simulink model "PMSM_DEE"  (R2023b)
settings: Solver=ode23t  StartTime=0.0  StopTime=0.4  RelTol=1e-3  EnableMultiTasking=on
libraries: powerlib_extras x3, spspowerguiLib x1
settings Model: Creator=Administrator  LastModifiedBy=Guoguo
settings SolverCC: AlgebraicLoopSolver=TrustRegion
settings DataIOCC: LimitDataPoints=on  SaveFormat=Array  SignalLoggingSaveFormat=ModelDataLogs  ReturnWorkspaceOutputs=off
settings OptimizationCC: InitFltsAndDblsToZero=on  LifeSpan=inf
settings DebuggingCC: SaveWithParameterizedLinksMsg=none  UnderspecifiedInitializationDetection=Classic  MergeDetectMultiDrivingBlocksExec=none  SolverPrmCheckMsg=warning  MultiTaskCondExecSysMsg=none  FcnCallInpInsideContextMsg=warning  UnconnectedInputMsg=warning  UnconnectedOutputMsg=warning  UnconnectedLineMsg=warning  SFUnexpectedBacktrackingDiag=warning  SFNoUnconditionalDefaultTransitionDiag=warning  SFExecutionAtInitializationDiag=none  ArithmeticOperatorsInVariantConditions=warning
settings HardwareCC: ProdBitPerPointer=32  ProdBitPerSizeT=32  ProdBitPerPtrDiffT=32  ProdLargestAtomicFloat=None  ProdIntDivRoundTo=Undefined  ProdEndianess=Unspecified  ProdWordSize=32  ProdHWDeviceType=32-bit Generic
settings ModelReferenceCC: PropagateSignalLabelsOutOfModel=off
settings SFSimCC: SimUseLocalCustomCode=off  CustomCodeUndefinedFunction=UseInterfaceOnly
settings RTWCC: RTWUseLocalCustomCode=off
settings CodeAppCC: StateflowObjectComments=on
settings GRTTargetCC: TargetFcnLib=ansi_tfl_tmw.mat  TargetLangStandard=C89/C90 (ANSI)  CombineOutputUpdateFcns=off  GRTInterface=on
settings ConfigComp: CovMetricSettings=dw  CovSaveCumulativeToWorkspaceVar=on  CovSaveSingleToWorkspaceVar=on  CovExternalEMLEnable=off  CovSFcnEnable=off

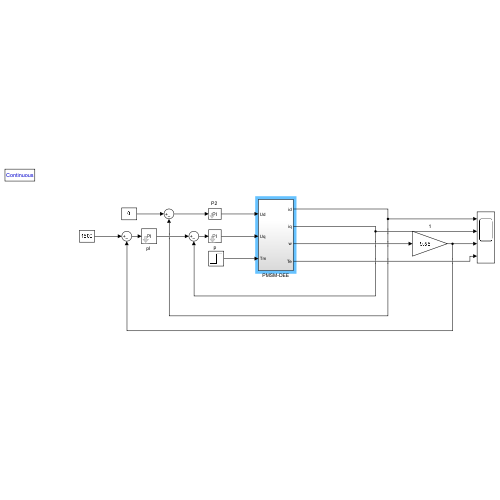
[thumbnail: Simulink's stored preview of the top-level diagram]
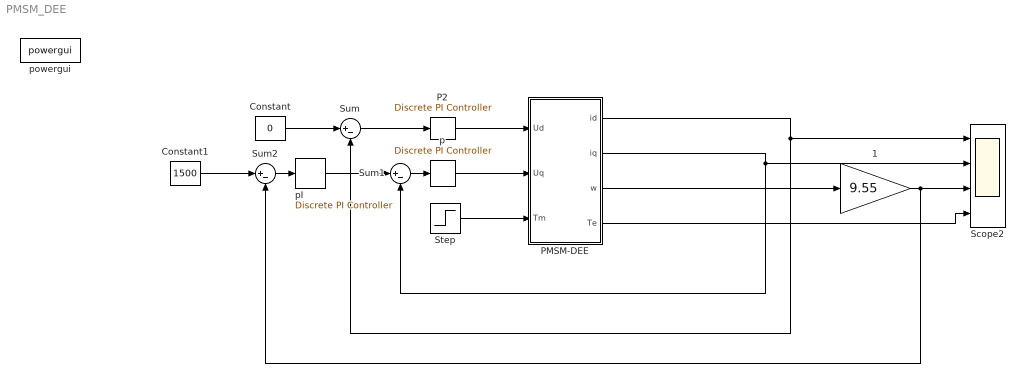
== system PMSM_DEE ==
  1 : Gain  Gain=9.55
  Constant : Constant  Value=0
  Constant1 : Constant  Value=1500
  "P2 " : powerlib_extras/Discrete  Control Blocks/Discrete PI Controller  Kp=21.25  Ki=7187.5  Par_Limits=[250 -250]  Init=0  Ts=50e-6
  PMSM-DEE : Subsystem
  Scope2 : Scope  NumInputPorts=4
  Step : Step  Time=0.2  After=10  SampleTime=0
  Sum : Sum  Inputs=|+-
  Sum1 : Sum  Inputs=|+-
  Sum2 : Sum  Inputs=|+-
  p : powerlib_extras/Discrete  Control Blocks/Discrete PI Controller  Kp=21.25  Ki=7187.5  Par_Limits=[300 -200]  Init=0  Ts=50e-6
  "pI " : powerlib_extras/Discrete  Control Blocks/Discrete PI Controller  Kp=0.16  Ki=10  Par_Limits=[30 -30]  Init=0  Ts=50e-6
  powergui : spspowerguiLib/powergui  SimulationMode=Continuous  SampleTime=50e-6  frequency=60  Iterations=50  frequencyindice=0  Pbase=100e6  ErrMax=1e-4  UnitsV=kV  UnitsW=MW  buscounter=0  FunctionMessages=off  echomessages=off  EnableUseOfTLC=off  CurrentSourceSwitches=on  DisableSnubberDevices=off  DisableRonSwitches=off  DisableVfSwitches=off  DisplayEquations=off  AutomaticDiscreteSolvers=off  SolverType=Tustin/Backward Euler (TBE)  Interpol=off  ExternalGateDelay=off  methode=off  Ts=0  x0status=blocks  SPID=off  SwTol=0  HookPort=off  NonlinearTolerance=1e-4  nMaxIteration=100  ContinueOnMaxIteration=off  RestoreLinks=warning  ResistiveCurrentMeasurement=off  Frange=[0:2:500]  Ylog=off  Xlog=on  ShowGrid=off  save=off  variable=ZData  structure=0  ZoomFFT=off  StartTime=0.0  cycles=1  DisplayStyle=1  fundamental=60  FreqAxis=off  MaxFrequency=1000  frequencyindicesteady=1  RmsSteady=1  display=off
  wires:
  Sum/1 -> "P2 "/1
  Sum1/1 -> p/1
  "pI "/1 -> Sum1/1
  Constant/1 -> Sum/1
  Sum2/1 -> "pI "/1
  1/1 -> Sum2/2, Scope2/3
  Constant1/1 -> Sum2/1
  PMSM-DEE/1(id) -> Sum/2, Scope2/1
  PMSM-DEE/2(iq) -> Sum1/2, Scope2/2
  p/1 -> PMSM-DEE/2(Uq)
  "P2 "/1 -> PMSM-DEE/1(Ud)
  PMSM-DEE/3(w) -> 1/1
  PMSM-DEE/4(Te) -> Scope2/4
  Step/1 -> PMSM-DEE/3(Tm)

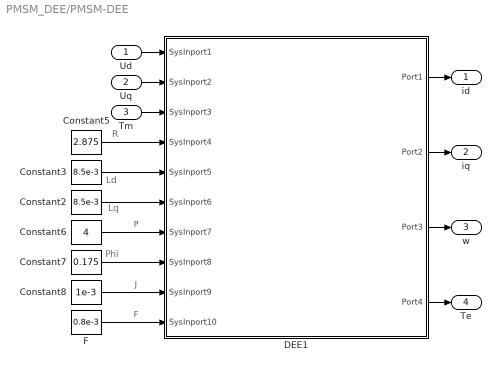
== system PMSM_DEE/PMSM-DEE ==
  note: Phi
  note: Lq
  note: Ld
  note: R
  Ud : Inport
  Uq : Inport  Port=2
  Tm : Inport  Port=3
  Constant2 : Constant  Value=8.5e-3
  Constant3 : Constant  Value=8.5e-3
  Constant5 : Constant  Value=2.875
  Constant6 : Constant  Value=4
  Constant7 : Constant  Value=0.175
  Constant8 : Constant  Value=1e-3
  DEE1 : Subsystem  mask(Differential Equation Editor (DEE)){}
      settings: OpenFcn=diffeqed
      mask Display: disp('Differential Equation\n Editor')
  F : Constant  Value=0.8e-3
  id : Outport
  iq : Outport  Port=2
  w : Outport  Port=3
  Te : Outport  Port=4
  wires:
  Constant5/1 -> DEE1/4(SysInport4)
  Constant3/1 -> DEE1/5(SysInport5)
  Constant2/1 -> DEE1/6(SysInport6)
  Constant6/1 -> DEE1/7(SysInport7)  "P"
  Constant7/1 -> DEE1/8(SysInport8)
  Constant8/1 -> DEE1/9(SysInport9)  "J"
  F/1 -> DEE1/10(SysInport10)  "F"
  Ud/1 -> DEE1/1(SysInport1)
  Uq/1 -> DEE1/2(SysInport2)
  DEE1/1(Port1) -> id/1
  Tm/1 -> DEE1/3(SysInport3)
  DEE1/2(Port2) -> iq/1
  DEE1/3(Port3) -> w/1
  DEE1/4(Port4) -> Te/1

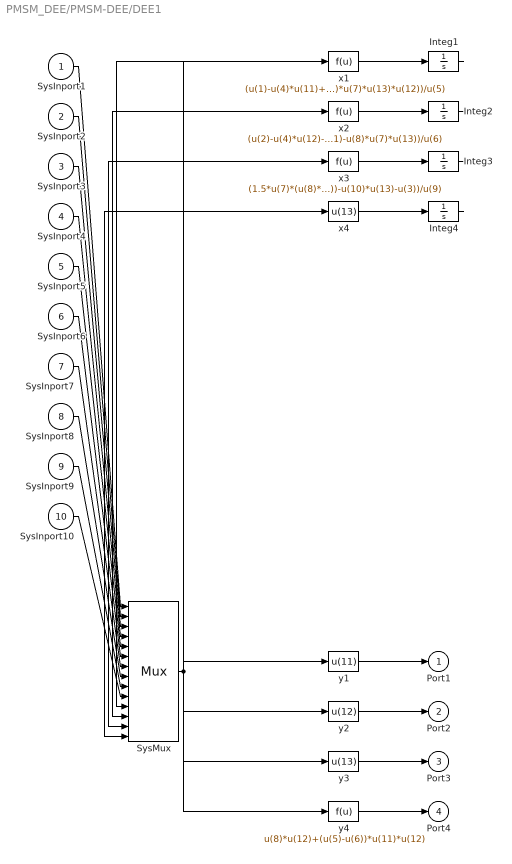
== system PMSM_DEE/PMSM-DEE/DEE1 ==
  SysInport1 : Inport
  SysInport2 : Inport  Port=2
  SysInport3 : Inport  Port=3
  SysInport4 : Inport  Port=4
  SysInport5 : Inport  Port=5
  SysInport6 : Inport  Port=6
  SysInport7 : Inport  Port=7
  SysInport8 : Inport  Port=8
  SysInport9 : Inport  Port=9
  SysInport10 : Inport  Port=10
  Integ{1..4} (4 alike) : Integrator
  SysMux : Mux  Inputs=14
  x1 : Fcn  Expr=(u(1)-u(4)*u(11)+u(6)*u(7)*u(13)*u(12))/u(5)
  x2 : Fcn  Expr=(u(2)-u(4)*u(12)-u(5)*u(7)*u(13)*u(11)-u(8)*u(7)*u(13))/u(6)
  x3 : Fcn  Expr=(1.5*u(7)*(u(8)*u(12)+(u(5)-u(6))*u(11)*u(12))-u(10)*u(13)-u(3))/u(9)
  x4 : Fcn  Expr=u(13)
  y1 : Fcn  Expr=u(11)
  y2 : Fcn  Expr=u(12)
  y3 : Fcn  Expr=u(13)
  y4 : Fcn  Expr=u(8)*u(12)+(u(5)-u(6))*u(11)*u(12)
  Port1 : Outport
  Port2 : Outport  Port=2
  Port3 : Outport  Port=3
  Port4 : Outport  Port=4
  wires:
  SysInport1/1 -> SysMux/1
  SysInport2/1 -> SysMux/2
  SysInport3/1 -> SysMux/3
  SysInport4/1 -> SysMux/4
  SysInport5/1 -> SysMux/5
  SysInport6/1 -> SysMux/6
  SysInport7/1 -> SysMux/7
  SysInport8/1 -> SysMux/8
  SysInport9/1 -> SysMux/9
  SysInport10/1 -> SysMux/10
  SysMux/1 -> x1/1, x2/1, x3/1, x4/1, y1/1, y2/1, y3/1, y4/1
  x1/1 -> Integ1/1
  Integ1/1 -> SysMux/11
  x2/1 -> Integ2/1
  Integ2/1 -> SysMux/12
  x3/1 -> Integ3/1
  Integ3/1 -> SysMux/13
  x4/1 -> Integ4/1
  Integ4/1 -> SysMux/14
  y1/1 -> Port1/1
  y2/1 -> Port2/1
  y3/1 -> Port3/1
  y4/1 -> Port4/1
